simulink model "Cuantificador2"  (R2013a)
settings: Solver=ode45  StartTime=0.0  StopTime=3.7874  RelTol=1e-3
settings Model: Creator=Alfonso  LastModifiedBy=Alfonso

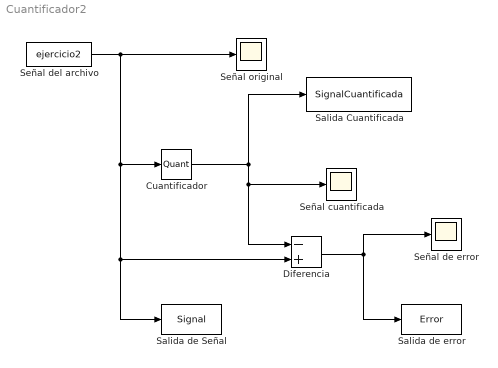
== system Cuantificador2 ==
  Cuantificador : Quantizer  QuantizationInterval=256
  Diferencia : Sum  Inputs=-+
  Salida Cuantificada : ToWorkspace  VariableName=SignalCuantificada  SampleTime=-1
  Salida de Señal : ToWorkspace  VariableName=Signal  SampleTime=-1
  Salida de error : ToWorkspace  VariableName=Error  SampleTime=-1
  Señal cuantificada : Scope
      settings: YMin=-10000  YMax=15000
  Señal de error : Scope
      settings: YMin=-150  YMax=150  SaveName=ScopeData2
  Señal del archivo : FromWorkspace  VariableName=ejercicio2  SampleTime=1/8000
  Señal original : Scope
      settings: YMin=-10000  YMax=15000
  wires:
  Señal del archivo/1 -> Salida de Señal/1, Diferencia/2, Cuantificador/1, Señal original/1
  Cuantificador/1 -> Diferencia/1, Señal cuantificada/1, Salida Cuantificada/1
  Diferencia/1 -> Señal de error/1, Salida de error/1
